simulink model "convertor_R2022b_cu_FromWorkspace"  (R2024b)
settings: Solver=VariableStepAuto  StartTime=0.0  StopTime=10.0  RelTol=1e-3
values from neighbouring files (symbols this model uses):
  Cv = 600e-6/3*m    (= 0.0004)    [de_la_gabi_bun.m]    (also in setup_convertor.m = 0.0016; setup_convertor_baiat.m; setup_convertor_bun_ultimul.m; setup_convertor_datele_mele.m)
  E = 12    [de_la_gabi_bun.m]    (also in setup_convertor.m; setup_convertor_baiat.m; setup_convertor_bun_ultimul.m; setup_convertor_datele_mele.m)
  Lv = 40e-3*3/m    (= 0.06)    [de_la_gabi_bun.m]    (also in setup_convertor.m = 0.015; setup_convertor_baiat.m; setup_convertor_bun_ultimul.m; setup_convertor_datele_mele.m)
  meas_rep = 13+ceil(n/2)    [de_la_gabi_bun.m]    (also in setup_convertor.m; setup_convertor_baiat.m; setup_convertor_bun_ultimul.m; setup_convertor_datele_mele.m)
  R = 15    [de_la_gabi_bun.m]    (also in setup_convertor.m; setup_convertor_baiat.m; setup_convertor_bun_ultimul.m; setup_convertor_datele_mele.m)
  rC = 0.2    [de_la_gabi_bun.m]    (also in setup_convertor.m; setup_convertor_baiat.m; setup_convertor_bun_ultimul.m; setup_convertor_datele_mele.m)
  rDS1 = 0.01    [de_la_gabi_bun.m]    (also in setup_convertor.m; setup_convertor_baiat.m; setup_convertor_bun_ultimul.m; setup_convertor_datele_mele.m)
  rDS2 = 0.01    [de_la_gabi_bun.m]    (also in setup_convertor.m; setup_convertor_baiat.m; setup_convertor_bun_ultimul.m; setup_convertor_datele_mele.m)
  rL = 10e-3    (= 0.01)    [de_la_gabi_bun.m]    (also in setup_convertor.m; setup_convertor_baiat.m; setup_convertor_bun_ultimul.m; setup_convertor_datele_mele.m)
  Ts = round(Ts*1e6)/1e6    [de_la_gabi_bun.m]    (also in setup_convertor.m; setup_convertor_baiat.m; setup_convertor_bun_ultimul.m; setup_convertor_datele_mele.m)
  umax = 0.98    [de_la_gabi_bun.m]    (also in setup_convertor.m; setup_convertor_baiat.m; setup_convertor_bun_ultimul.m; setup_convertor_datele_mele.m)
  umin = 0    [de_la_gabi_bun.m]    (also in setup_convertor.m; setup_convertor_baiat.m; setup_convertor_bun_ultimul.m; setup_convertor_datele_mele.m)
  whtn_pow_in = 1e-11*(Ts*1e4)/2    (= 7.30769230769e-13)    [de_la_gabi_bun.m]    (also in setup_convertor.m = 1.20588235294e-12; setup_convertor_baiat.m; setup_convertor_bun_ultimul.m; setup_convertor_datele_mele.m = 8.75e-13)
  whtn_pow_out = 1e-7*E*(Ts*1e4/50)*(1+(50*u_star)*(u_star-0.15))/3    (= 1.68223076923e-09)    [de_la_gabi_bun.m]    (also in setup_convertor.m = 1.96414117647e-08; setup_convertor_baiat.m; setup_convertor_bun_ultimul.m; setup_convertor_datele_mele.m = 2.912e-09)
  whtn_seed_in = 23341+m+2*n    (= 23345)    [de_la_gabi_bun.m]    (also in setup_convertor.m = 23365; setup_convertor_baiat.m; setup_convertor_bun_ultimul.m; setup_convertor_datele_mele.m = 23347)
  whtn_seed_out = 23342-m-2*n    (= 23338)    [de_la_gabi_bun.m]    (also in setup_convertor.m = 23318; setup_convertor_baiat.m; setup_convertor_bun_ultimul.m; setup_convertor_datele_mele.m = 23336)
  whtn_Ts_in = Ts*2    (= 2.92307692308e-05)    [de_la_gabi_bun.m]    (also in setup_convertor.m = 4.82352941176e-05; setup_convertor_baiat.m; setup_convertor_bun_ultimul.m; setup_convertor_datele_mele.m = 3.5e-05)
  whtn_Ts_out = Ts*2    (= 2.92307692308e-05)    [de_la_gabi_bun.m]    (also in setup_convertor.m = 4.82352941176e-05; setup_convertor_baiat.m; setup_convertor_bun_ultimul.m; setup_convertor_datele_mele.m = 3.5e-05)
  x0_slx = [(-1)^(n+1)*E/R,E/3/(1-u_star)]    [de_la_gabi_bun.m]    (also in setup_convertor.m; setup_convertor_baiat.m; setup_convertor_bun_ultimul.m; setup_convertor_datele_mele.m)
  ymax = 1/(1-u_star)*E*2    (= 29.8136645963)    [de_la_gabi_bun.m]    (also in setup_convertor.m = 48.9795918367; setup_convertor_baiat.m; setup_convertor_bun_ultimul.m; setup_convertor_datele_mele.m = 31.5789473684)
  ymin = 0    [de_la_gabi_bun.m]    (also in setup_convertor.m; setup_convertor_baiat.m; setup_convertor_bun_ultimul.m; setup_convertor_datele_mele.m)
libraries: simulink x2
settings Model: Creator=Miruna  LastModifiedBy=Miruna

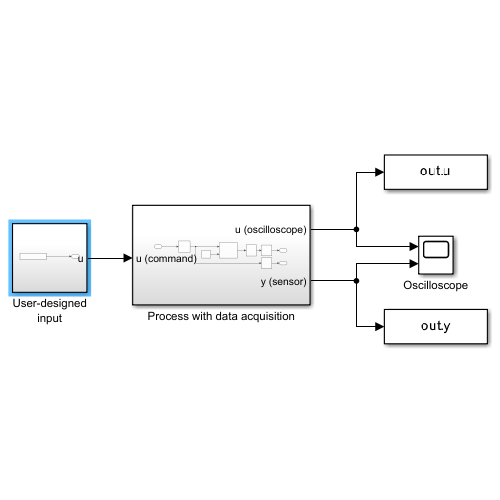
[thumbnail: Simulink's stored preview of the top-level diagram]
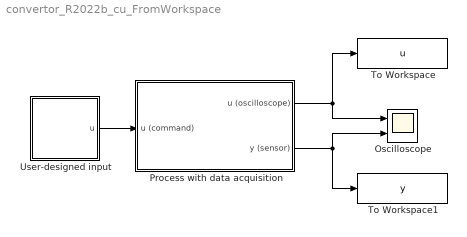
== system convertor_R2022b_cu_FromWorkspace ==
  Oscilloscope : Scope  NumInputPorts=2
  Process with data acquisition : Subsystem
  To Workspace : ToWorkspace  VariableName=u  SampleTime=Ts
  To Workspace1 : ToWorkspace  VariableName=y  SampleTime=Ts
  User-designed input : Subsystem
  wires:
  Process with data acquisition/1(u (oscilloscope)) -> Oscilloscope/1, To Workspace/1
  User-designed input/1(u) -> Process with data acquisition/1(u (command))
  Process with data acquisition/2(y (sensor)) -> Oscilloscope/2, To Workspace1/1

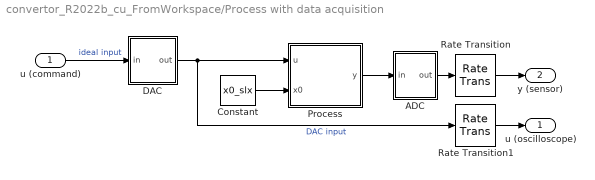
== system convertor_R2022b_cu_FromWorkspace/Process with data acquisition ==
  u (command) : Inport
  ADC : Subsystem
  Constant : Constant  Value=x0_slx
  DAC : Subsystem
  Process : Subsystem
  Rate Transition : RateTransition  OutPortSampleTime=Ts*meas_rep
  Rate Transition1 : RateTransition  OutPortSampleTime=Ts*meas_rep
  u (oscilloscope) : Outport
  y (sensor) : Outport  Port=2
  wires:
  Constant/1 -> Process/2(x0)
  u (command)/1 -> DAC/1(in)  "ideal input"
  Process/1(y) -> ADC/1(in)
  ADC/1(out) -> Rate Transition/1
  DAC/1(out) -> Process/1(u), Rate Transition1/1  "DAC input"
  Rate Transition/1 -> y (sensor)/1
  Rate Transition1/1 -> u (oscilloscope)/1

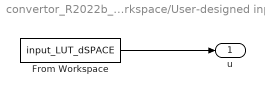
== system convertor_R2022b_cu_FromWorkspace/User-designed input ==
  From Workspace : FromWorkspace  VariableName=input_LUT_dSPACE  SampleTime=Ts
  u : Outport
  wires:
  From Workspace/1 -> u/1

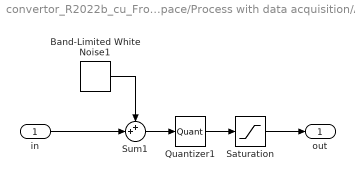
== system convertor_R2022b_cu_FromWorkspace/Process with data acquisition/ADC ==
  in : Inport
  Band-Limited White Noise1 : simulink/Sources/Band-Limited White Noise  Cov=[whtn_pow_out]  Ts=whtn_Ts_out  seed=[whtn_seed_out]
  Quantizer1 : Quantizer  QuantizationInterval=q_out
  Saturation : Saturate  UpperLimit=ymax  LowerLimit=ymin
  Sum1 : Sum  Inputs=++|
  out : Outport
  wires:
  Quantizer1/1 -> Saturation/1
  Sum1/1 -> Quantizer1/1
  in/1 -> Sum1/2
  Band-Limited White Noise1/1 -> Sum1/1
  Saturation/1 -> out/1

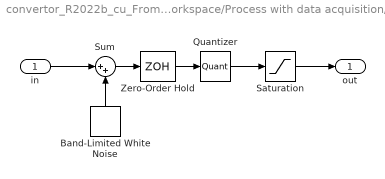
== system convertor_R2022b_cu_FromWorkspace/Process with data acquisition/DAC ==
  in : Inport
  Band-Limited White Noise : simulink/Sources/Band-Limited White Noise  Cov=[whtn_pow_in]  Ts=whtn_Ts_in  seed=[whtn_seed_in]
  Quantizer : Quantizer  QuantizationInterval=q_in
  Saturation : Saturate  UpperLimit=umax  LowerLimit=umin
  Sum : Sum  Inputs=|++
  Zero-Order Hold : ZeroOrderHold  SampleTime=-1
  out : Outport
  wires:
  Quantizer/1 -> Saturation/1
  Sum/1 -> Zero-Order Hold/1
  in/1 -> Sum/1
  Band-Limited White Noise/1 -> Sum/2
  Zero-Order Hold/1 -> Quantizer/1
  Saturation/1 -> out/1

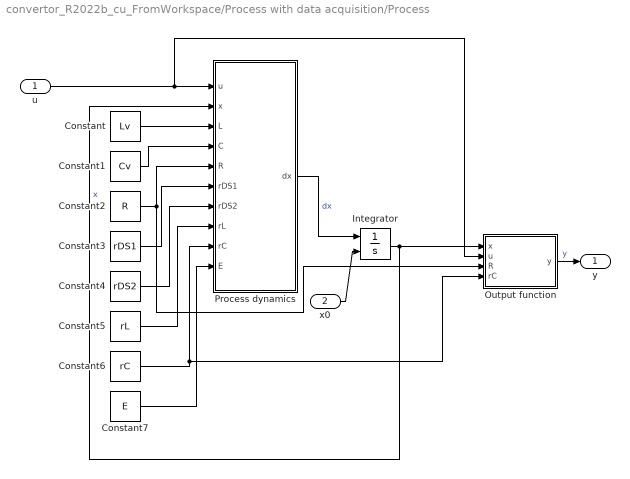
== system convertor_R2022b_cu_FromWorkspace/Process with data acquisition/Process ==
  u : Inport
  x0 : Inport  Port=2
  Constant : Constant  Value=Lv
  Constant1 : Constant  Value=Cv
  Constant2 : Constant  Value=R
  Constant3 : Constant  Value=rDS1
  Constant4 : Constant  Value=rDS2
  Constant5 : Constant  Value=rL
  Constant6 : Constant  Value=rC
  Constant7 : Constant  Value=E
  Integrator : Integrator  InitialConditionSource=external
  Output function : MATLAB Function  TreatAsAtomicUnit=on
  Process dynamics : MATLAB Function  TreatAsAtomicUnit=on
  y : Outport
  wires:
  u/1 -> Output function/2(u), Process dynamics/1(u)
  Process dynamics/1(dx) -> Integrator/1  "dx"
  Integrator/1 -> Output function/1(x), Process dynamics/2(x)  "x"
  Output function/1(y) -> y/1  "y"
  x0/1 -> Integrator/2
  Constant/1 -> Process dynamics/3(L)
  Constant1/1 -> Process dynamics/4(C)
  Constant2/1 -> Output function/3(R), Process dynamics/5(R)
  Constant3/1 -> Process dynamics/6(rDS1)
  Constant4/1 -> Process dynamics/7(rDS2)
  Constant5/1 -> Process dynamics/8(rL)
  Constant6/1 -> Output function/4(rC), Process dynamics/9(rC)
  Constant7/1 -> Process dynamics/10(E)

== matlab function convertor_R2022b_cu_FromWorkspace/Process with data acquisition/Process/Process dynamics ==
  data: u input; dx output; x input; L input; C input; R input; rDS1 input; rDS2 input; rL input; rC input; E input
function dx = fcn(u,x,L,C,R,rDS1,rDS2,rL,rC,E)

r_aux = rL + rDS2 + rC*R/(R+rC); 

Aon = [-(rL+rDS1)/L,0;0,-1/(R+rC)/C];
Aoff = [-r_aux/L,-R/(R+rC)/L;R/(R+rC)/C,-1/(R+rC)/C];
Bon = [1/L;0];
Boff = [1/L;0];

dx = (u*Aon+(1-u)*Aoff)*x+(u*Bon+(1-u)*Boff)*E;

== matlab function convertor_R2022b_cu_FromWorkspace/Process with data acquisition/Process/Output function ==
  data: y output; x input; u input; R input; rC input
function y = fcn(x,u,R,rC)

Con = [0,R/(R+rC)];
Coff = [rC*R/(R+rC),R/(R+rC)];
y = (u*Con+(1-u)*Coff)*x;

end
